simulink model "PI_Controller"  (R2020a)
settings: Solver=VariableStepAuto  StartTime=0.0  StopTime=120  RelTol=1e-3
undefined symbols (not defined in the file or in its folder): Ki, Kp
settings Model: DataDictionary=DD23.sldd  Creator=HP  LastModifiedBy=HP
settings DataIOCC: SaveOutput=off  SaveTime=off

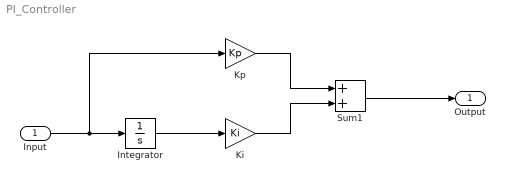
== system PI_Controller ==
  Input : Inport  OutDataTypeStr=double  PortDimensions=1  SampleTime=0
  Integrator : Integrator
  Ki : Gain  Gain=Ki
  Kp : Gain  Gain=Kp
  Sum1 : Sum
  Output : Outport  OutDataTypeStr=double  PortDimensions=1  SampleTime=0
  wires:
  Integrator/1 -> Ki/1
  Ki/1 -> Sum1/2
  Input/1 -> Integrator/1, Kp/1
  Kp/1 -> Sum1/1
  Sum1/1 -> Output/1
